simulink model "CAES_Compression"  (R2022a)
settings: Solver=VariableStepAuto  StartTime=0.0  StopTime=200  RelTol=1e-3
values from neighbouring files (symbols this model uses):
  Dc = 0    [CAES_Parameters.m]
  eps_hx1 = 0.8785    [CAES_Parameters.m]
  eps_hx2 = 0.8    [CAES_Parameters.m]
  eps_hx3 = 0.8    [CAES_Parameters.m]
  eps_hx4 = 0.8    [CAES_Parameters.m]
  Hc = 12.957    [CAES_Parameters.m]
  Kcd = 0.214    [CAES_Parameters.m]
  Kci = 0.1485    [CAES_Parameters.m]
  Kcp = 0.4147    [CAES_Parameters.m]
  lmax = 1.15    [CAES_Parameters.m]
  lmin = 0.6-0.5    (= 0.1)    [CAES_Parameters.m]
  R = 0.04    [CAES_Parameters.m]
  tau_hx1 = 12    [CAES_Parameters.m]
  tau_hx2 = 12    [CAES_Parameters.m]
  tau_hx3 = 12    [CAES_Parameters.m]
  tau_hx4 = 12    [CAES_Parameters.m]
  tauCD = 0.2    [CAES_Parameters.m]
  tauCP = 0.02    [CAES_Parameters.m]
  tauIGV = 0.2    [CAES_Parameters.m]
  Tci1 = 283.15    [CAES_Parameters.m]
  Thxin = 298.7    [CAES_Parameters.m]
  umax = 1.2+0.3    (= 1.5)    [CAES_Parameters.m]
  umin = 0    [CAES_Parameters.m]
libraries: slpidlib x1, spspowerguiLib x1
settings Model: Creator=xiaojs20  LastModifiedBy=xiaojs20

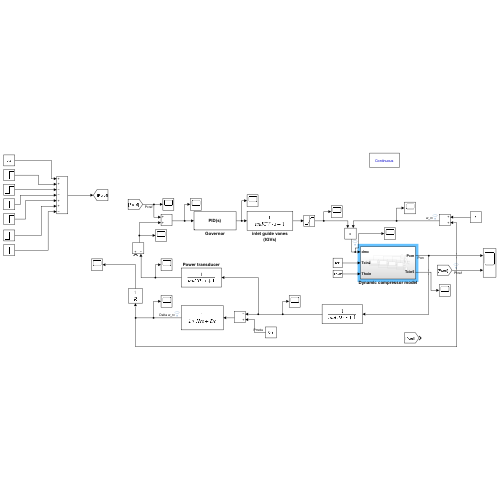
[thumbnail: Simulink's stored preview of the top-level diagram]
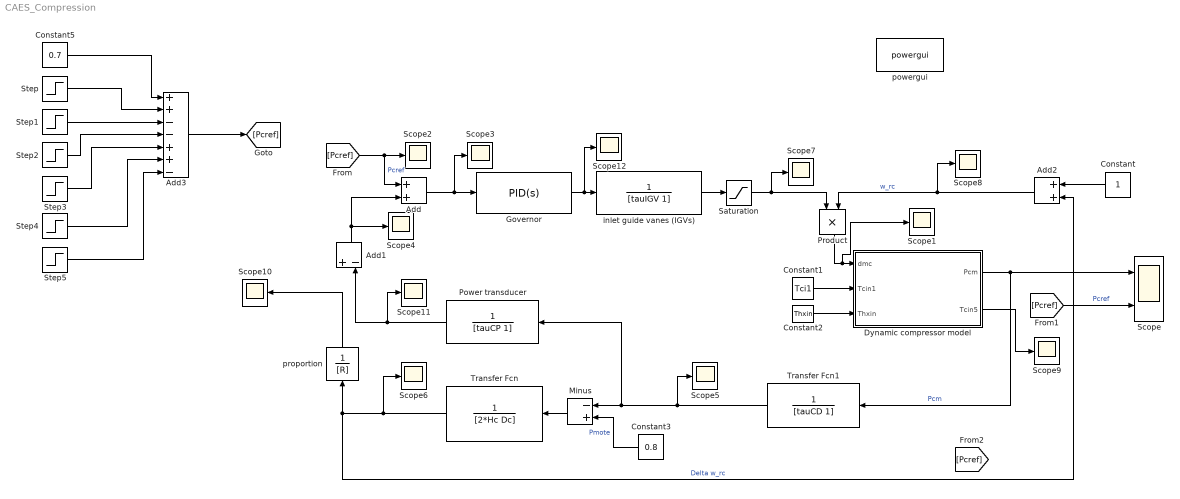
== system CAES_Compression ==
  Add : Sum
  Add1 : Sum  Inputs=+-
  Add2 : Sum
  Add3 : Sum  Inputs=++--++-
  Constant : Constant
  Constant1 : Constant  Value=Tci1
  Constant2 : Constant  Value=Thxin
  Constant3 : Constant  Value=0.8
  Constant5 : Constant  Value=0.7
  Dynamic compressor model : Subsystem
  Governor : slpidlib/PID Controller  Controller=PID  Form=Parallel  TimeDomain=Continuous-time  UseExternalTs=off  SampleTime=-1  IntegratorMethod=Forward Euler  FilterMethod=Forward Euler  ControllerParametersSource=internal  P=Kcp  I=Kci  UseKiTs=off  D=Kcd  N=100  UseFilter=on  TunerSelectOption=Transfer Function Based (PID Tuner App)  InitialConditionSource=internal  InitialConditionForIntegrator=0  InitialConditionForFilter=0  DifferentiatorICPrevScaledInput=0  ExternalReset=none  TrackingMode=off  Kt=1  LimitOutput=off  SatLimitsSource=internal  UpperSaturationLimit=umax  LowerSaturationLimit=umin  LinearizeAsGain=on  AntiWindupMode=none  Kb=1  POutMin=[]  POutMax=[]  IOutMin=[]  IOutMax=[]  DOutMin=[]  DOutMax=[]  NOutMin=[]  NOutMax=[]  SumOutMin=[]  SumOutMax=[]  SaturationOutMin=[]  SaturationOutMax=[]  PParamMin=[]  PParamMax=[]  IParamMin=[]  IParamMax=[]  DParamMin=[]  DParamMax=[]  NParamMin=[]  NParamMax=[]  KbParamMin=[]  KbParamMax=[]  KtParamMin=[]  KtParamMax=[]  KbOutMin=[]  KbOutMax=[]  KtOutMin=[]  KtOutMax=[]  IntegratorOutMin=[]  IntegratorOutMax=[]  FilterOutMin=[]  FilterOutMax=[]  SumI1OutMin=[]  SumI1OutMax=[]  SumI2OutMin=[]  SumI2OutMax=[]  SumI3OutMin=[]  SumI3OutMax=[]  SumI4OutMin=[]  SumI4OutMax=[]  SumDOutMin=[]  SumDOutMax=[]  DifferentiatorOutMin=[]  DifferentiatorOutMax=[]  FilterDiffOutCoefMin=[]  FilterDiffOutCoefMax=[]  ReciprocalOutMin=[]  ReciprocalOutMax=[]  SumDenOutMin=[]  SumDenOutMax=[]  SumNumOutMin=[]  SumNumOutMax=[]  DivideOutMin=[]  DivideOutMax=[]  UdiffTsProdOutMin=[]  UdiffTsProdOutMax=[]  NTsProdOutMin=[]  NTsProdOutMax=[]  UintegralTsProdOutMin=[]  UintegralTsProdOutMax=[]  UngainTsProdOutMin=[]  UngainTsProdOutMax=[]  IntegratorContinuousStateAttributes=''  IntegratorStateMustResolveToSignalObject=off  IntegratorRTWStateStorageClass=Auto  FilterContinuousStateAttributes=''  FilterStateMustResolveToSignalObject=off  FilterRTWStateStorageClass=Auto  ParallelPVariant=InternalParameters  IdealPVariant=Disabled  IVariant=InternalParameters  DVariant=InternalParameters  IntegratorVariant=Continuous  SatVariant=Disabled  AWVariant=Passthrough  PCopyVariant=Disabled  TRVariant=Disabled  FdbkBlocksVariant=Forward  IdealPFdbkVariant=Disabled  SatFdbkVariant=Disabled  DerivativeFilterVariant=ContFilter  NVariant=InternalParameters  NCopyVariant=Disabled  FilterICVariant=InternalICsFilter  IntegratorICVariant=InternalICs  ExternalResetVariant=Disabled  TRSumVariant=Passthrough  SumFdbkVariant=Disabled  SumVariant=Sum_PID  TsampFilterVariant=InternalTs  TsampNgainVariant=Passthrough  TsampIntegralVariant=Passthrough  ExternalSaturationOutDataTypeStr=Inherit: Same as second input  aMode=0
  Minus : Sum  Inputs=-+
  Power transducer : TransferFcn  Denominator=[tauCP 1]
  Product : Product
  Saturation : Saturate  UpperLimit=lmax  LowerLimit=lmin
  Scope : Scope  NumInputPorts=2
  Scope{1..12} (12 alike) : Scope
  Step : Step  Time=5  After=0.3  SampleTime=0  ZeroCross=off
  Step1 : Step  Time=30  After=0.3  SampleTime=0  ZeroCross=off
  Step2 : Step  Time=60  After=0.1  SampleTime=0  ZeroCross=off
  Step3 : Step  Time=80  After=0.1  SampleTime=0  ZeroCross=off
  Step4 : Step  Time=120  After=0.5  SampleTime=0  ZeroCross=off
  Step5 : Step  Time=140  After=0.5  SampleTime=0  ZeroCross=off
  Transfer Fcn : TransferFcn  Denominator=[2*Hc Dc]
  Transfer Fcn1 : TransferFcn  Denominator=[tauCD 1]
  inlet guide vanes (IGVs) : TransferFcn  Denominator=[tauIGV 1]
  powergui : spspowerguiLib/powergui  Priority=1  SimulationMode=Continuous  SampleTime=50e-6  frequency=60  Iterations=50  frequencyindice=60  Pbase=100e6  ErrMax=1e-4  UnitsV=kV  UnitsW=MW  buscounter=0  FunctionMessages=off  echomessages=off  EnableUseOfTLC=off  CurrentSourceSwitches=off  DisableSnubberDevices=off  DisableRonSwitches=off  DisableVfSwitches=off  DisplayEquations=off  AutomaticDiscreteSolvers=off  SolverType=Tustin/Backward Euler (TBE)  Interpol=off  ExternalGateDelay=off  methode=off  Ts=100  x0status=blocks  SPID=on  SwTol=0  HookPort=off  NonlinearTolerance=1e-4  nMaxIteration=100  ContinueOnMaxIteration=off  RestoreLinks=warning  ResistiveCurrentMeasurement=off  Frange=[0:2:500]  Ylog=off  Xlog=on  ShowGrid=off  save=off  variable=ZData  structure=0  ZoomFFT=off  StartTime=0.0  cycles=1  DisplayStyle=1  fundamental=60  FreqAxis=off  MaxFrequency=1000  frequencyindicesteady=1  RmsSteady=1  display=off
  proportion : TransferFcn  Denominator=[R]
  wires:
  Add3/1 -> [Pcref]
  Step/1 -> Add3/2
  Constant5/1 -> Add3/1
  Step1/1 -> Add3/3
  Step2/1 -> Add3/4
  Step3/1 -> Add3/5
  Step4/1 -> Add3/6
  Step5/1 -> Add3/7
  Add/1 -> Scope3/1, Governor/1
  [Pcref] -> Scope2/1, Add/1  "Pcref"
  Add1/1 -> Add/2, Scope4/1
  proportion/1 -> Scope10/1
  Transfer Fcn/1 -> Scope6/1, proportion/1, Add2/2  "Delta w_rc"
  Power transducer/1 -> Scope11/1, Add1/2
  Transfer Fcn1/1 -> Scope5/1, Power transducer/1, Minus/1
  Minus/1 -> Transfer Fcn/1
  Governor/1 -> Scope12/1, inlet guide vanes (IGVs)/1
  inlet guide vanes (IGVs)/1 -> Saturation/1
  Saturation/1 -> Scope7/1, Product/1
  Constant/1 -> Add2/1
  Add2/1 -> Scope8/1, Product/2  "w_rc"
  Product/1 -> Scope1/1, Dynamic compressor model/1(dmc)
  Constant1/1 -> Dynamic compressor model/2(Tcin1)
  Constant2/1 -> Dynamic compressor model/3(Thxin)
  Dynamic compressor model/1(Pcm) -> Transfer Fcn1/1, Scope/1  "Pcm"
  Constant3/1 -> Minus/2  "Pmote"
  [Pcref] -> Scope/2  "Pcref"
  Dynamic compressor model/2(Tcin5) -> Scope9/1

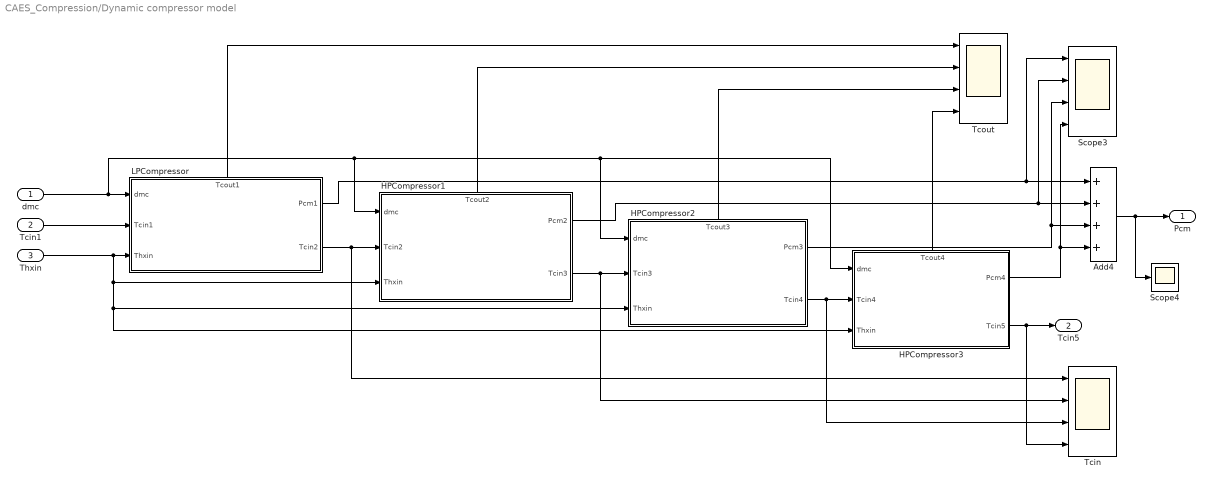
== system CAES_Compression/Dynamic compressor model ==
  dmc : Inport
  Tcin1 : Inport  Port=2
  Thxin : Inport  Port=3
  Add4 : Sum  Inputs=++++
  HPCompressor1 : Subsystem
      settings: PortSchema="{\"entries\":[{\"content\":{\"sides\":[{\"content\":{\"connectorIds\":[\"In1\",\"In2\",\"In3\"]},\"type\":\"ConnectorPlacement.EquallySpacedRectSide\",\"uuid\":\"57af89d3-241d-4c70-8baa-ac60b98bf504\"},{\"content\":{\"connectorIds\":[\"Out1\",\"Out2\"],\"side\":\"RIGHT\"},\"type\":\"ConnectorPlacement.EquallySpacedRectSide\",\"uuid\":\"d2cff914-a280-4cce-988c-97fa844b2264\"},{\"content\":{\"connectorIds\":[\"Out3\"],\"side\":\"TOP\"},\"type\":\"ConnectorPlacement.EquallySpacedRectSide\",\"uuid\":\"6571594b-71b5-4a3e-8683-a0578b05fbde\"}]},\"type\":\"ConnectorPlacement.EquallySpacedConnector\",\"uuid\":\"24807979-4286-4f7f-927b-e4e6b18eb233\"}],\"packageUris\":[\"http://schema.mathworks.com/mf0/Connector/R2020b\"],\"version\":\"1.0\"}"
  HPCompressor2 : Subsystem
      settings: PortSchema="{\"entries\":[{\"content\":{\"sides\":[{\"content\":{\"connectorIds\":[\"In1\",\"In2\",\"In3\"]},\"type\":\"ConnectorPlacement.EquallySpacedRectSide\",\"uuid\":\"57af89d3-241d-4c70-8baa-ac60b98bf504\"},{\"content\":{\"connectorIds\":[\"Out1\",\"Out2\"],\"side\":\"RIGHT\"},\"type\":\"ConnectorPlacement.EquallySpacedRectSide\",\"uuid\":\"d2cff914-a280-4cce-988c-97fa844b2264\"},{\"content\":{\"connectorIds\":[\"Out3\"],\"side\":\"TOP\"},\"type\":\"ConnectorPlacement.EquallySpacedRectSide\",\"uuid\":\"6571594b-71b5-4a3e-8683-a0578b05fbde\"}]},\"type\":\"ConnectorPlacement.EquallySpacedConnector\",\"uuid\":\"24807979-4286-4f7f-927b-e4e6b18eb233\"}],\"packageUris\":[\"http://schema.mathworks.com/mf0/Connector/R2020b\"],\"version\":\"1.0\"}"
  HPCompressor3 : Subsystem
      settings: PortSchema="{\"entries\":[{\"content\":{\"sides\":[{\"content\":{\"connectorIds\":[\"In1\",\"In2\",\"In3\"]},\"type\":\"ConnectorPlacement.EquallySpacedRectSide\",\"uuid\":\"57af89d3-241d-4c70-8baa-ac60b98bf504\"},{\"content\":{\"connectorIds\":[\"Out1\",\"Out2\"],\"side\":\"RIGHT\"},\"type\":\"ConnectorPlacement.EquallySpacedRectSide\",\"uuid\":\"d2cff914-a280-4cce-988c-97fa844b2264\"},{\"content\":{\"connectorIds\":[\"Out3\"],\"side\":\"TOP\"},\"type\":\"ConnectorPlacement.EquallySpacedRectSide\",\"uuid\":\"6571594b-71b5-4a3e-8683-a0578b05fbde\"}]},\"type\":\"ConnectorPlacement.EquallySpacedConnector\",\"uuid\":\"24807979-4286-4f7f-927b-e4e6b18eb233\"}],\"packageUris\":[\"http://schema.mathworks.com/mf0/Connector/R2020b\"],\"version\":\"1.0\"}"
  LPCompressor : Subsystem
      settings: PortSchema="{\"entries\":[{\"content\":{\"sides\":[{\"content\":{\"connectorIds\":[\"In1\",\"In2\",\"In3\"]},\"type\":\"ConnectorPlacement.EquallySpacedRectSide\",\"uuid\":\"57af89d3-241d-4c70-8baa-ac60b98bf504\"},{\"content\":{\"connectorIds\":[\"Out1\",\"Out2\"],\"side\":\"RIGHT\"},\"type\":\"ConnectorPlacement.EquallySpacedRectSide\",\"uuid\":\"d2cff914-a280-4cce-988c-97fa844b2264\"},{\"content\":{\"connectorIds\":[\"Out3\"],\"side\":\"TOP\"},\"type\":\"ConnectorPlacement.EquallySpacedRectSide\",\"uuid\":\"6571594b-71b5-4a3e-8683-a0578b05fbde\"}]},\"type\":\"ConnectorPlacement.EquallySpacedConnector\",\"uuid\":\"24807979-4286-4f7f-927b-e4e6b18eb233\"}],\"packageUris\":[\"http://schema.mathworks.com/mf0/Connector/R2020b\"],\"version\":\"1.0\"}"
  Scope3 : Scope  NumInputPorts=4
  Scope4 : Scope
  Tcin : Scope  NumInputPorts=4
  Tcout : Scope  NumInputPorts=4
  Pcm : Outport
  Tcin5 : Outport  Port=2
  wires:
  LPCompressor/1(Pcm1) -> Add4/1, Scope3/1
  Tcin1/1 -> LPCompressor/2(Tcin1)
  Add4/1 -> Scope4/1, Pcm/1
  Thxin/1 -> HPCompressor3/3(Thxin), HPCompressor2/3(Thxin), HPCompressor1/3(Thxin), LPCompressor/3(Thxin)
  dmc/1 -> HPCompressor1/1(dmc), HPCompressor2/1(dmc), HPCompressor3/1(dmc), LPCompressor/1(dmc)
  HPCompressor2/1(Pcm3) -> Scope3/3, Add4/3
  HPCompressor1/1(Pcm2) -> Add4/2, Scope3/2
  HPCompressor3/2(Tcin5) -> Tcin/4, Tcin5/1
  HPCompressor3/1(Pcm4) -> Scope3/4, Add4/4
  HPCompressor1/2(Tcin3) -> Tcin/2, HPCompressor2/2(Tcin3)
  LPCompressor/2(Tcin2) -> Tcin/1, HPCompressor1/2(Tcin2)
  HPCompressor2/2(Tcin4) -> Tcin/3, HPCompressor3/2(Tcin4)
  HPCompressor3/3(Tcout4) -> Tcout/4
  HPCompressor2/3(Tcout3) -> Tcout/3
  HPCompressor1/3(Tcout2) -> Tcout/2
  LPCompressor/3(Tcout1) -> Tcout/1

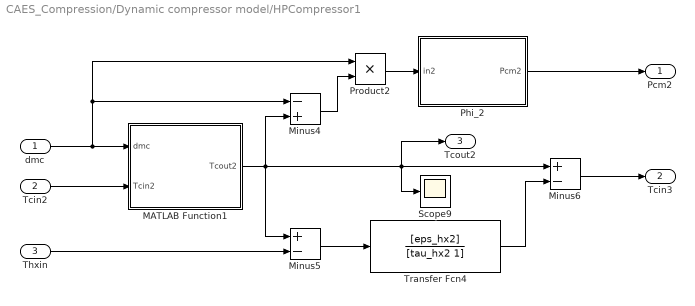
== system CAES_Compression/Dynamic compressor model/HPCompressor1 ==
  dmc : Inport
  Tcin2 : Inport  Port=2
  Thxin : Inport  Port=3
  MATLAB Function1 : MATLAB Function  TreatAsAtomicUnit=on
  Minus4 : Sum  Inputs=-+
  Minus5 : Sum  Inputs=+-
  Minus6 : Sum  Inputs=+-
  Phi_2 : MATLAB Function  TreatAsAtomicUnit=on
  Product2 : Product
  Scope9 : Scope
  Transfer Fcn4 : TransferFcn  Numerator=[eps_hx2]  Denominator=[tau_hx2 1]
  Pcm2 : Outport
  Tcin3 : Outport  Port=2
  Tcout2 : Outport  Port=3
  wires:
  Thxin/1 -> Minus5/2
  dmc/1 -> MATLAB Function1/1(dmc), Product2/1, Minus4/1
  Phi_2/1(Pcm2) -> Pcm2/1
  Minus5/1 -> Transfer Fcn4/1
  Minus4/1 -> Product2/2
  Product2/1 -> Phi_2/1(in2)
  Minus6/1 -> Tcin3/1
  Transfer Fcn4/1 -> Minus6/2
  Tcin2/1 -> MATLAB Function1/2(Tcin2)
  MATLAB Function1/1(Tcout2) -> Minus5/1, Tcout2/1, Scope9/1, Minus6/1, Minus4/2

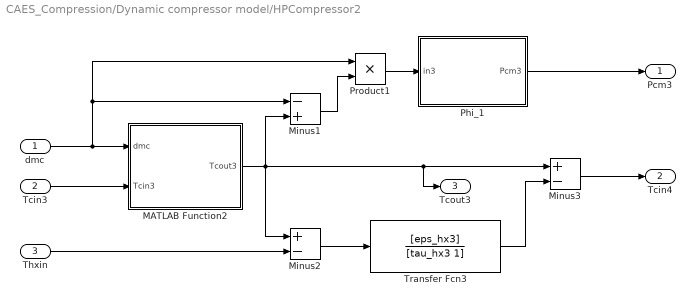
== system CAES_Compression/Dynamic compressor model/HPCompressor2 ==
  dmc : Inport
  Tcin3 : Inport  Port=2
  Thxin : Inport  Port=3
  MATLAB Function2 : MATLAB Function  TreatAsAtomicUnit=on
  Minus1 : Sum  Inputs=-+
  Minus2 : Sum  Inputs=+-
  Minus3 : Sum  Inputs=+-
  Phi_1 : MATLAB Function  TreatAsAtomicUnit=on
  Product1 : Product
  Transfer Fcn3 : TransferFcn  Numerator=[eps_hx3]  Denominator=[tau_hx3 1]
  Pcm3 : Outport
  Tcin4 : Outport  Port=2
  Tcout3 : Outport  Port=3
  wires:
  Minus1/1 -> Product1/2
  Product1/1 -> Phi_1/1(in3)
  Minus3/1 -> Tcin4/1
  Transfer Fcn3/1 -> Minus3/2
  Phi_1/1(Pcm3) -> Pcm3/1
  Minus2/1 -> Transfer Fcn3/1
  dmc/1 -> MATLAB Function2/1(dmc), Product1/1, Minus1/1
  Thxin/1 -> Minus2/2
  Tcin3/1 -> MATLAB Function2/2(Tcin3)
  MATLAB Function2/1(Tcout3) -> Minus2/1, Tcout3/1, Minus3/1, Minus1/2

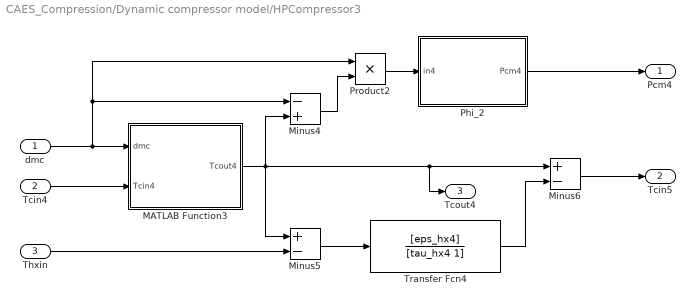
== system CAES_Compression/Dynamic compressor model/HPCompressor3 ==
  dmc : Inport
  Tcin4 : Inport  Port=2
  Thxin : Inport  Port=3
  MATLAB Function3 : MATLAB Function  TreatAsAtomicUnit=on
  Minus4 : Sum  Inputs=-+
  Minus5 : Sum  Inputs=+-
  Minus6 : Sum  Inputs=+-
  Phi_2 : MATLAB Function  TreatAsAtomicUnit=on
  Product2 : Product
  Transfer Fcn4 : TransferFcn  Numerator=[eps_hx4]  Denominator=[tau_hx4 1]
  Pcm4 : Outport
  Tcin5 : Outport  Port=2
  Tcout4 : Outport  Port=3
  wires:
  dmc/1 -> MATLAB Function3/1(dmc), Product2/1, Minus4/1
  Minus5/1 -> Transfer Fcn4/1
  Phi_2/1(Pcm4) -> Pcm4/1
  Minus6/1 -> Tcin5/1
  Thxin/1 -> Minus5/2
  Transfer Fcn4/1 -> Minus6/2
  Tcin4/1 -> MATLAB Function3/2(Tcin4)
  Minus4/1 -> Product2/2
  Product2/1 -> Phi_2/1(in4)
  MATLAB Function3/1(Tcout4) -> Minus5/1, Tcout4/1, Minus6/1, Minus4/2

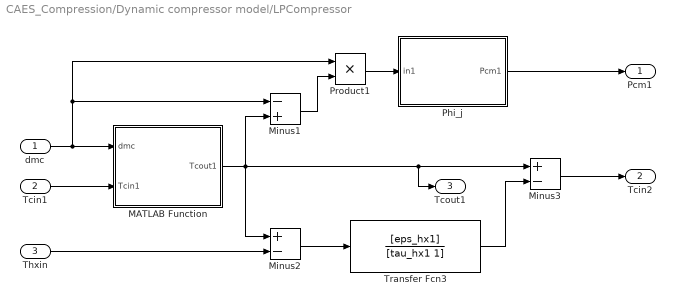
== system CAES_Compression/Dynamic compressor model/LPCompressor ==
  dmc : Inport
  Tcin1 : Inport  Port=2
  Thxin : Inport  Port=3
  MATLAB Function : MATLAB Function  TreatAsAtomicUnit=on
  Minus1 : Sum  Inputs=-+
  Minus2 : Sum  Inputs=+-
  Minus3 : Sum  Inputs=+-
  Phi_j : MATLAB Function  TreatAsAtomicUnit=on
  Product1 : Product
  Transfer Fcn3 : TransferFcn  Numerator=[eps_hx1]  Denominator=[tau_hx1 1]
  Pcm1 : Outport
  Tcin2 : Outport  Port=2
  Tcout1 : Outport  Port=3
  wires:
  MATLAB Function/1(Tcout1) -> Minus2/1, Tcout1/1, Minus3/1, Minus1/2
  Transfer Fcn3/1 -> Minus3/2
  dmc/1 -> Product1/1, Minus1/1, MATLAB Function/1(dmc)
  Tcin1/1 -> MATLAB Function/2(Tcin1)
  Minus3/1 -> Tcin2/1
  Product1/1 -> Phi_j/1(in1)
  Minus1/1 -> Product1/2
  Phi_j/1(Pcm1) -> Pcm1/1
  Minus2/1 -> Transfer Fcn3/1
  Thxin/1 -> Minus2/2

== matlab function CAES_Compression/Dynamic compressor model/LPCompressor/MATLAB Function ==
  data: dmc input; Tcout1 output; Tcin1 input
function Tcout1 = Gamma1(dmc,Tcin1)
    eta_ci1=0.8200; 

    gamma=1.4;
    a11=6.6686; a12=2.9654;
    g=(gamma-1)/gamma;
    pi_c1=a11*sqrt(1-dmc/a12);
    Gamma1=1+((pi_c1^g)-1)/eta_ci1;
    Tcout1=Tcin1*Gamma1;
end

== matlab function CAES_Compression/Dynamic compressor model/HPCompressor2/MATLAB Function2 ==
  data: dmc input; Tcout3 output; Tcin3 input
function Tcout3 = Gamma3(dmc,Tcin3)
    eta_ci3=0.9023;
    gamma=1.4;
    a21=2.8817; a22=2.9654;
    g=(gamma-1)/gamma;
    pi_c3=a21*sqrt(1-dmc/a22);
    Gamma2=1+((pi_c3^g)-1)/eta_ci3;
    Tcout3=Tcin3*Gamma2;
end

== matlab function CAES_Compression/Dynamic compressor model/HPCompressor3/MATLAB Function3 ==
  data: dmc input; Tcout4 output; Tcin4 input
function Tcout4 = Gamma4(dmc,Tcin4)
    eta_ci4=0.9097;
    gamma=1.4;
    a21=2.8817; a22=2.9654;
    g=(gamma-1)/gamma;
    pi_c4=a21*sqrt(1-dmc/a22);
    Gamma2=1+((pi_c4^g)-1)/eta_ci4;
    Tcout4=Tcin4*Gamma2;
end

== matlab function CAES_Compression/Dynamic compressor model/LPCompressor/Phi_j ==
  data: in1 input; Pcm1 output
function Pcm1 = Phi1(in1)
    cp=1.055;
    dmco=108; %kg/s
    eta_cm1=0.99;
    Pcmo=58.7;

    Phi1=(cp*dmco)/(1e3*eta_cm1*Pcmo);
    Pcm1=in1*Phi1;
end

== matlab function CAES_Compression/Dynamic compressor model/HPCompressor1/Phi_2 ==
  data: in2 input; Pcm2 output
function Pcm2 = Phi2(in2)
    cp=1.055;
    dmco=108; %kg/s
    eta_cm2=0.99;
    Pcmo=58.7;

    Phi2=(cp*dmco)/(1e3*eta_cm2*Pcmo);
    Pcm2=in2*Phi2;
end

== matlab function CAES_Compression/Dynamic compressor model/HPCompressor2/Phi_1 ==
  data: in3 input; Pcm3 output
function Pcm3 = Phi3(in3)
    cp=1.055;
    dmco=108; %kg/s
    eta_cm3=0.99;
    Pcmo=58.7;

    Phi3=(cp*dmco)/(1e3*eta_cm3*Pcmo);
    Pcm3=in3*Phi3;
end

== matlab function CAES_Compression/Dynamic compressor model/HPCompressor3/Phi_2 ==
  data: in4 input; Pcm4 output
function Pcm4 = Phi4(in4)
    cp=1.055;
    dmco=108; %kg/s
    eta_cm4=0.99;
    Pcmo=58.7;

    Phi4=(cp*dmco)/(1e3*eta_cm4*Pcmo);
    Pcm4=in4*Phi4;
end

== matlab function CAES_Compression/Dynamic compressor model/HPCompressor1/MATLAB Function1 ==
  data: dmc input; Tcout2 output; Tcin2 input
function Tcout2 = Gamma2(dmc,Tcin2)
    eta_ci2=0.9115;
    gamma=1.4;
    a21=2.8817; a22=2.9654;
    g=(gamma-1)/gamma;
    pi_c1=a21*sqrt(1-dmc/a22);
    Gamma2=1+((pi_c1^g)-1)/eta_ci2;
    Tcout2=Tcin2*Gamma2;
end
